simulink model "Res_1"  (R2018b)
settings: Solver=VariableStepAuto  StartTime=0.0  StopTime=60  RelTol=1e-3
values from neighbouring files (symbols this model uses):
  b = 0.06    [result_1.m]
  J = 0.5    [result_1.m]
settings Model: Creator=makha  LastModifiedBy=makha

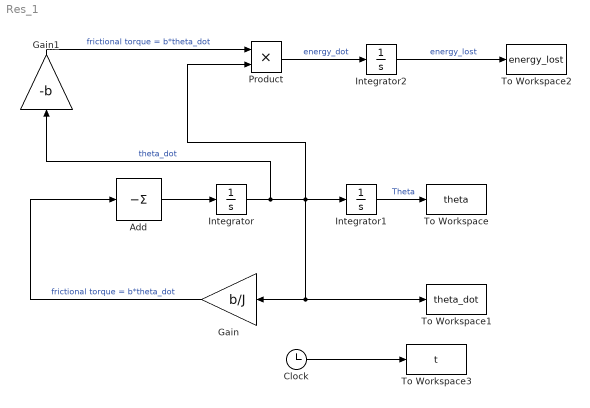
== system Res_1 ==
  Add : Sum  Inputs=-
  Clock : Clock
  Gain : Gain  Gain=b/J
  Gain1 : Gain  Gain=-b
  Integrator : Integrator  InitialCondition=40
  Integrator1 : Integrator
  Integrator2 : Integrator
  Product : Product
  To Workspace : ToWorkspace  VariableName=theta  SampleTime=-1
  To Workspace1 : ToWorkspace  VariableName=theta_dot  SampleTime=-1
  To Workspace2 : ToWorkspace  VariableName=energy_lost  SampleTime=-1
  To Workspace3 : ToWorkspace  VariableName=t  SampleTime=-1
  wires:
  Gain/1 -> Add/1  "frictional torque = b*theta_dot"
  Add/1 -> Integrator/1
  Integrator/1 -> Product/2, Integrator1/1, To Workspace1/1, Gain/1, Gain1/1  "theta_dot"
  Integrator1/1 -> To Workspace/1  "Theta"
  Product/1 -> Integrator2/1  "energy_dot"
  Integrator2/1 -> To Workspace2/1  "energy_lost"
  Clock/1 -> To Workspace3/1
  Gain1/1 -> Product/1  "frictional torque = b*theta_dot"
